simulink model "FIR_Filter"  (R2020a)
settings: Solver=VariableStepAuto  StartTime=0.0  StopTime=10.0  RelTol=1e-3
settings Model: Creator=USER  LastModifiedBy=USER
settings DataIOCC: SaveOutput=off  SaveTime=off

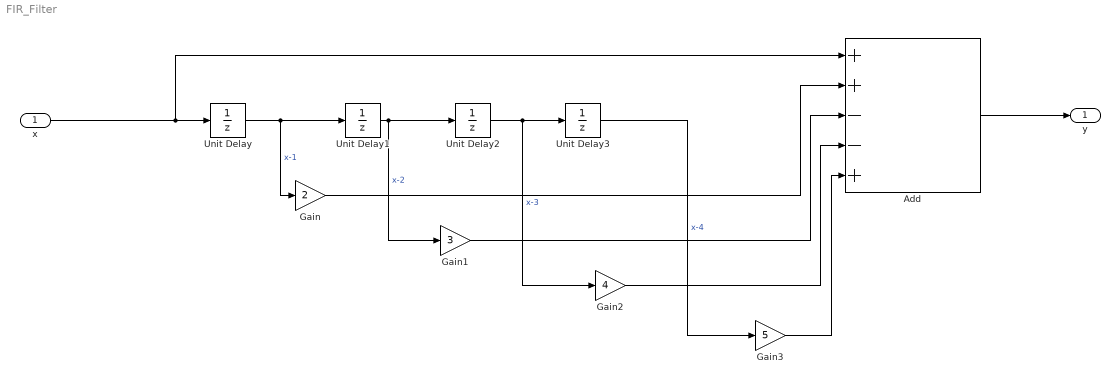
== system FIR_Filter ==
  x : Inport  OutDataTypeStr=double  PortDimensions=1  SampleTime=[0,1]
  Add : Sum  Inputs=++--+
  Gain : Gain  Gain=2
  Gain1 : Gain  Gain=3
  Gain2 : Gain  Gain=4
  Gain3 : Gain  Gain=5
  Unit Delay{,1..3} (4 alike) : UnitDelay  SampleTime=-1  HasFrameUpgradeWarning=on
  y : Outport  OutDataTypeStr=double  PortDimensions=1  SampleTime=[0,1]
  wires:
  x/1 -> Unit Delay/1, Add/1
  Unit Delay3/1 -> Gain3/1  "x-4"
  Add/1 -> y/1
  Gain/1 -> Add/2
  Unit Delay2/1 -> Gain2/1, Unit Delay3/1  "x-3"
  Gain1/1 -> Add/3
  Unit Delay/1 -> Gain/1, Unit Delay1/1  "x-1"
  Gain2/1 -> Add/4
  Unit Delay1/1 -> Gain1/1, Unit Delay2/1  "x-2"
  Gain3/1 -> Add/5
